simulink model "Lab1_parameter_estimation_student_M2"  (R2024b)
settings: Solver=FixedStepAuto  StartTime=0  StopTime=20  FixedStep=0.01  RelTol=1e-3
values from neighbouring files (symbols this model uses):
  motor_B = 0.0001    [Lab1_motor_params_student.m]
  motor_Efficiency = 0.8    [Lab1_motor_params_student.m]
  motor_J = 0.001    [Lab1_motor_params_student.m]
  motor_Ke = 0.05    [Lab1_motor_params_student.m]
  motor_L = 0.0877797954    [Lab1_motor_params_student.m]
  motor_R = 0.92384    [Lab1_motor_params_student.m]
libraries: simulink x1
settings Model: Creator=tanawatp  LastModifiedBy=acer
settings RTWCC: GPUComputeCapability=3.5

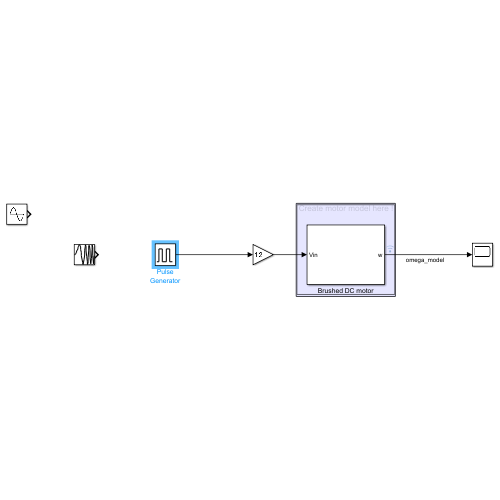
[thumbnail: Simulink's stored preview of the top-level diagram]
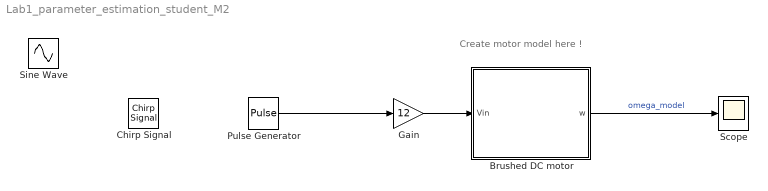
== system Lab1_parameter_estimation_student_M2 ==
  note: Create motor model here !
  Brushed DC motor : Subsystem
  Chirp Signal : simulink/Sources/Chirp Signal  f1=0  T=20  f2=1
  Gain : Gain  Gain=12
  Pulse Generator : DiscretePulseGenerator  PulseType=Time based  PulseWidth=50
  Scope : Scope
  Sine Wave : Sin  Frequency=0.2  SampleTime=0
  wires:
  Brushed DC motor/1(w) -> Scope/1  "omega_model"
  Gain/1 -> Brushed DC motor/1(Vin)
  Pulse Generator/1 -> Gain/1

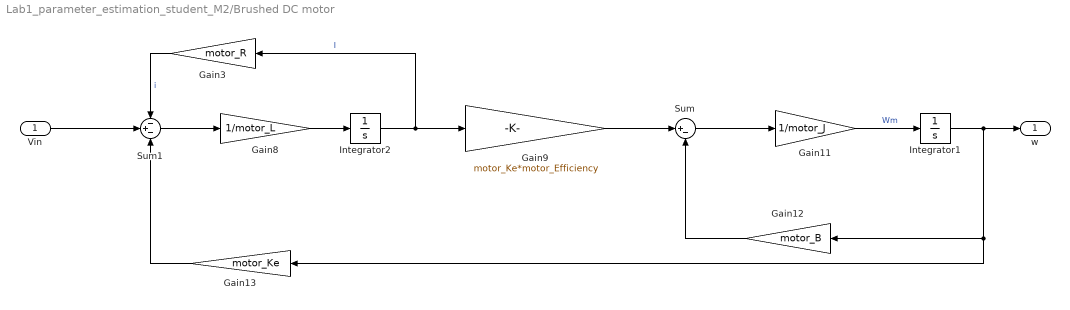
== system Lab1_parameter_estimation_student_M2/Brushed DC motor ==
  Vin : Inport
  Gain11 : Gain  Gain=1/motor_J
  Gain12 : Gain  Gain=motor_B
  Gain13 : Gain  Gain=motor_Ke
  Gain3 : Gain  Gain=motor_R
  Gain8 : Gain  Gain=1/motor_L
  Gain9 : Gain  Gain=motor_Ke*motor_Efficiency
  Integrator1 : Integrator
  Integrator2 : Integrator
  Sum : Sum  Inputs=|+-
  Sum1 : Sum  Inputs=-+-
  w : Outport
  wires:
  Gain9/1 -> Sum/1
  Sum/1 -> Gain11/1
  Gain12/1 -> Sum/2
  Gain11/1 -> Integrator1/1  "Wm"
  Integrator1/1 -> Gain12/1, Gain13/1, w/1
  Vin/1 -> Sum1/2
  Gain3/1 -> Sum1/1  "i"
  Gain13/1 -> Sum1/3
  Sum1/1 -> Gain8/1
  Gain8/1 -> Integrator2/1
  Integrator2/1 -> Gain3/1, Gain9/1  "I"
